simulink model "QUESTION2_4"  (R2021a)
settings: Solver=VariableStepAuto  StartTime=0.0  StopTime=50  RelTol=1e-3
settings Model: Creator=user  LastModifiedBy=user

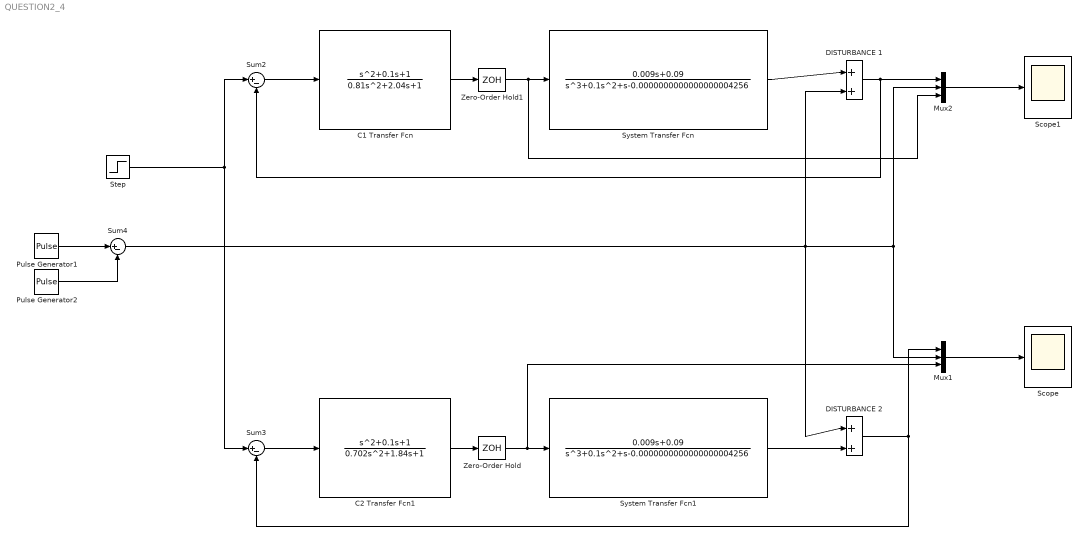
== system QUESTION2_4 ==
  C1 Transfer Fcn : TransferFcn  Numerator=[1 0.1 1]  Denominator=[0.81 2.04 1]
  C2 Transfer Fcn1 : TransferFcn  Numerator=[1 0.1 1]  Denominator=[0.702 1.84 1]
  DISTURBANCE 1 : Sum  Inputs=|++
  DISTURBANCE 2 : Sum  Inputs=|++
  Mux1 : Mux  Inputs=3
  Mux2 : Mux  Inputs=3
  Pulse Generator1 : DiscretePulseGenerator  PulseType=Time based  Period=1  PhaseDelay=20  SampleTime=-1
  Pulse Generator2 : DiscretePulseGenerator  PulseType=Time based  Period=1  PhaseDelay=23  SampleTime=-1
  Scope : Scope
  Scope1 : Scope
  Step : Step  SampleTime=0
  Sum2 : Sum  Inputs=|+-
  Sum3 : Sum  Inputs=|+-
  Sum4 : Sum  Inputs=|+-
  System Transfer Fcn : TransferFcn  Numerator=[0.009 0.09]  Denominator=[1 0.1 1 -0.0000000000000000004256]
  System Transfer Fcn1 : TransferFcn  Numerator=[0.009 0.09]  Denominator=[1 0.1 1 -0.0000000000000000004256]
  Zero-Order Hold : ZeroOrderHold  SampleTime=-1
  Zero-Order Hold1 : ZeroOrderHold  SampleTime=-1
  wires:
  Step/1 -> Sum3/1, Sum2/1
  Mux1/1 -> Scope/1
  Sum2/1 -> C1 Transfer Fcn/1
  Sum3/1 -> C2 Transfer Fcn1/1
  Pulse Generator1/1 -> Sum4/1
  Pulse Generator2/1 -> Sum4/2
  Sum4/1 -> Mux2/2, Mux1/2, DISTURBANCE 2/1, DISTURBANCE 1/2
  Mux2/1 -> Scope1/1
  System Transfer Fcn/1 -> DISTURBANCE 1/1
  DISTURBANCE 1/1 -> Mux2/1, Sum2/2
  DISTURBANCE 2/1 -> Sum3/2, Mux1/1
  System Transfer Fcn1/1 -> DISTURBANCE 2/2
  C2 Transfer Fcn1/1 -> Zero-Order Hold/1
  Zero-Order Hold/1 -> Mux1/3, System Transfer Fcn1/1
  C1 Transfer Fcn/1 -> Zero-Order Hold1/1
  Zero-Order Hold1/1 -> Mux2/3, System Transfer Fcn/1
